simulink model "PARTAGE_last"  (Simulink 7.5)
settings: Solver=ode45  StartTime=0.0  StopTime=inf  RelTol=1e-3
settings Model: Creator=paris  LastModifiedBy=paris

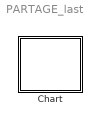
== system PARTAGE_last ==
  Chart : Stateflow chart  TreatAsAtomicUnit=on

== stateflow chart Chart ==
  state MODEL_ACTIVITE_SITUEE [parallel]
    settings: executionOrder=1
    state franchissement_VAG
      state Sortie_Virage
      state Fin_Gestion_Courbe
      state VAG_JAC_SVD
        state Entree_Virage
        state Approche_Virage
        state Debut_Gestion_Courbe
        MODEL_ACTIVITE_SITUEE.franchissement_VAG.VAG_JAC_SVD.Approche_Virage -> MODEL_ACTIVITE_SITUEE.franchissement_VAG.VAG_JAC_SVD.Entree_Virage : [ml.distPtA<=10]
        MODEL_ACTIVITE_SITUEE.franchissement_VAG.VAG_JAC_SVD.Entree_Virage -> MODEL_ACTIVITE_SITUEE.franchissement_VAG.VAG_JAC_SVD.Debut_Gestion_Courbe : [ml.distPtA<=0.01]
        (default) -> MODEL_ACTIVITE_SITUEE.franchissement_VAG.VAG_JAC_SVD.Approche_Virage
      state Pas_Code
      (junction 74) -> VAG_JAC_SVD [order 1] : [ml.distPtA<=50 && ml.distPtC>=0]
      MODEL_ACTIVITE_SITUEE.franchissement_VAG.Fin_Gestion_Courbe -> MODEL_ACTIVITE_SITUEE.franchissement_VAG.Sortie_Virage : [ml.distPtC<=0.01]
      MODEL_ACTIVITE_SITUEE.franchissement_VAG.VAG_JAC_SVD.Debut_Gestion_Courbe -> MODEL_ACTIVITE_SITUEE.franchissement_VAG.Fin_Gestion_Courbe : [ml.distPtB<=0.01]
      (junction 74) -> MODEL_ACTIVITE_SITUEE.franchissement_VAG.Pas_Code [order 2]
      (default) -> (junction 74)
    state Debut_Situation/
    state franchissement_VAD
      state Sortie_Virage
      state Fin_Gestion_Courbe
      state VAD_JAC_SVG
        state Entree_Virage
        state Approche_Virage
        state Debut_Gestion_Courbe
        MODEL_ACTIVITE_SITUEE.franchissement_VAD.VAD_JAC_SVG.Approche_Virage -> MODEL_ACTIVITE_SITUEE.franchissement_VAD.VAD_JAC_SVG.Entree_Virage : [ml.distPtA<=10]
        MODEL_ACTIVITE_SITUEE.franchissement_VAD.VAD_JAC_SVG.Entree_Virage -> MODEL_ACTIVITE_SITUEE.franchissement_VAD.VAD_JAC_SVG.Debut_Gestion_Courbe : [ml.distPtA<=0.01]
        (default) -> MODEL_ACTIVITE_SITUEE.franchissement_VAD.VAD_JAC_SVG.Approche_Virage
      state Pas_Code
      (junction 75) -> VAD_JAC_SVG [order 1] : [ml.distPtA<=50 && ml.distPtC>=0]
      MODEL_ACTIVITE_SITUEE.franchissement_VAD.Fin_Gestion_Courbe -> MODEL_ACTIVITE_SITUEE.franchissement_VAD.Sortie_Virage : [ml.distPtC<=0.01]
      MODEL_ACTIVITE_SITUEE.franchissement_VAD.VAD_JAC_SVG.Debut_Gestion_Courbe -> MODEL_ACTIVITE_SITUEE.franchissement_VAD.Fin_Gestion_Courbe : [ml.distPtB<=0.01]
      (junction 75) -> MODEL_ACTIVITE_SITUEE.franchissement_VAD.Pas_Code [order 2]
      (default) -> (junction 75)
    state Gestion_obstacle
      state Depassement
        state Approche
        state Imminent
        state Debut_Depassement
        state Fin_Depassement
        MODEL_ACTIVITE_SITUEE.Gestion_obstacle.Depassement.Approche -> MODEL_ACTIVITE_SITUEE.Gestion_obstacle.Depassement.Imminent [order 1] : [ml.cligno==-1]
        MODEL_ACTIVITE_SITUEE.Gestion_obstacle.Depassement.Approche -> Debut_Depassement [order 2] : [ml.progression_SV==1]
        MODEL_ACTIVITE_SITUEE.Gestion_obstacle.Depassement.Imminent -> Debut_Depassement : [ml.progression_SV==1]
        Debut_Depassement -> Fin_Depassement : [ml.etat_obstacle==0]
        (default) -> MODEL_ACTIVITE_SITUEE.Gestion_obstacle.Depassement.Approche
      state Approche_Obstacle
      state Gestion_Interaction_ContreSens
        state Debut_Interaction
        state Fin_Interaction
        state Approche
        state Imminent
        Debut_Interaction -> Fin_Interaction : [ml.etat_obstacle==0]
        MODEL_ACTIVITE_SITUEE.Gestion_obstacle.Gestion_Interaction_ContreSens.Approche -> MODEL_ACTIVITE_SITUEE.Gestion_obstacle.Gestion_Interaction_ContreSens.Imminent [order 1] : [ml.tlc<=1 || ml.ttc<=2]
        MODEL_ACTIVITE_SITUEE.Gestion_obstacle.Gestion_Interaction_ContreSens.Imminent -> Debut_Interaction : [ml.progression_SV==1]
        MODEL_ACTIVITE_SITUEE.Gestion_obstacle.Gestion_Interaction_ContreSens.Approche -> Debut_Interaction [order 2] : [ml.progression_SV==1]
      state Gestion_Obstacle_Fixe
        state Debut_Gestion_Obstacle
        state Fin_Gestion_Obstacle
        state Imminent
        state Approche
        Debut_Gestion_Obstacle -> Fin_Gestion_Obstacle : [ml.etat_obstacle==0]
        MODEL_ACTIVITE_SITUEE.Gestion_obstacle.Gestion_Obstacle_Fixe.Imminent -> Debut_Gestion_Obstacle : [ml.progression_SV==1]
        (default) -> MODEL_ACTIVITE_SITUEE.Gestion_obstacle.Gestion_Obstacle_Fixe.Approche
        MODEL_ACTIVITE_SITUEE.Gestion_obstacle.Gestion_Obstacle_Fixe.Approche -> Debut_Gestion_Obstacle [order 2] : [ml.progression_SV==1]
        MODEL_ACTIVITE_SITUEE.Gestion_obstacle.Gestion_Obstacle_Fixe.Approche -> MODEL_ACTIVITE_SITUEE.Gestion_obstacle.Gestion_Obstacle_Fixe.Imminent [order 1] : [ml.tlc<=1 || ml.ttc<=2]
      Approche_Obstacle -> Depassement [order 1] : [ml.sensCirculation_obstacle==21 || ml.type_obstacle==30]
      (default) -> Approche_Obstacle [order 2]
      Approche_Obstacle -> Gestion_Interaction_ContreSens [order 2] : [ml.sensCirculation_obstacle==22 && ml.type_obstacle<>30]
      (default) -> MODEL_ACTIVITE_SITUEE.Gestion_obstacle.Gestion_Interaction_ContreSens.Approche [order 1]
      Approche_Obstacle -> Gestion_Obstacle_Fixe [order 3] : [ml.sensCirculation==20]
    state Fin_Situation
    (default) -> Debut_Situation
    Debut_Situation -> franchissement_VAG [order 2] : [(ml.type_infrastructure==60 || ml.type_infrastructure==61)]
    (junction 73) -> Fin_Situation : [ml.type_infrastructure==62]
    Debut_Situation -> franchissement_VAD [order 3] : [ml.type_infrastructure==63 || ml.type_infrastructure==64]
    Debut_Situation -> Gestion_obstacle [order 1] : [ml.etat_obstacle>0]
    franchissement_VAD -> (junction 73)
    Fin_Situation -> Debut_Situation
    franchissement_VAG -> (junction 73)
    Fin_Depassement -> (junction 71)
    Fin_Interaction -> (junction 71)
    Fin_Gestion_Obstacle -> (junction 71)
    (junction 71) -> Fin_Situation : [ml.etat_obstacle==0]
    MODEL_ACTIVITE_SITUEE.franchissement_VAD.Sortie_Virage -> Fin_Situation
    MODEL_ACTIVITE_SITUEE.franchissement_VAG.Sortie_Virage -> Fin_Situation
  state MANOEUVRE_SV [parallel]
    settings: executionOrder=2
    state Conduite_Dans_Voie
    state SORTIE_VOIE
      state SVG
        state HORS_VOIE
          state Recentration
          state Excentration
          MANOEUVRE_SV.SORTIE_VOIE.SVG.HORS_VOIE.Excentration -> MANOEUVRE_SV.SORTIE_VOIE.SVG.HORS_VOIE.Recentration : [ml.progression_SV==-1]
        state RSV
        MANOEUVRE_SV.SORTIE_VOIE.SVG.RSV -> MANOEUVRE_SV.SORTIE_VOIE.SVG.HORS_VOIE.Excentration : [ml.progression_SV==1]
        (default) -> MANOEUVRE_SV.SORTIE_VOIE.SVG.RSV
      state SVD
        state HORS_VOIE
          state Recentration
          state Excentration
          MANOEUVRE_SV.SORTIE_VOIE.SVD.HORS_VOIE.Excentration -> MANOEUVRE_SV.SORTIE_VOIE.SVD.HORS_VOIE.Recentration : [ml.progression_SV==-1]
        state RSV
        (default) -> MANOEUVRE_SV.SORTIE_VOIE.SVD.RSV
        MANOEUVRE_SV.SORTIE_VOIE.SVD.RSV -> MANOEUVRE_SV.SORTIE_VOIE.SVD.HORS_VOIE.Excentration : [ml.progression_SV==1]
    (default) -> MANOEUVRE_SV.Conduite_Dans_Voie
    MANOEUVRE_SV.SORTIE_VOIE.SVD.HORS_VOIE.Recentration -> MANOEUVRE_SV.Conduite_Dans_Voie : [ml.etat_SV==0]
    MANOEUVRE_SV.Conduite_Dans_Voie -> SVD [order 2] : [ml.lateralisation_SV==1 && in(Risque_Sortie_Voie.SV_Imminente)]
    MANOEUVRE_SV.SORTIE_VOIE.SVG.HORS_VOIE.Recentration -> MANOEUVRE_SV.Conduite_Dans_Voie : [ml.etat_SV==0]
    MANOEUVRE_SV.Conduite_Dans_Voie -> SVG [order 1] : [ml.lateralisation_SV==-1 && in(Risque_Sortie_Voie.SV_Imminente)]
  state Jugement_Adequation_Comportement [parallel]
    settings: executionOrder=3
    state Defaut_Maitrise
    state Sortie_Voie_Legitime
    state Conduite_Dans_Voie
    state Optimisation_Trajectoire
    (junction 70) -> Optimisation_Trajectoire [order 3] : [in(MODEL_ACTIVITE_SITUEE.franchissement_VAG.VAG_JAC_SVD) && in(MANOEUVRE_SV.SORTIE_VOIE.SVD)]
    (default) -> Jugement_Adequation_Comportement.Conduite_Dans_Voie
    Jugement_Adequation_Comportement.Conduite_Dans_Voie -> (junction 70) : [in(Risque_Sortie_Voie.SV_Imminente) || in(Risque_Sortie_Voie.SV_Effective)]
    (junction 70) -> Optimisation_Trajectoire [order 5] : [in(MODEL_ACTIVITE_SITUEE.franchissement_VAD.VAD_JAC_SVG) && in(MANOEUVRE_SV.SORTIE_VOIE.SVG) ]
    (junction 70) -> Sortie_Voie_Legitime [order 1] : [ml.etat_obstacle==1]
    (junction 70) -> Optimisation_Trajectoire [order 2] : [(in(MODEL_ACTIVITE_SITUEE.franchissement_VAG.VAG_JAC_SVD) || in(MODEL_ACTIVITE_SITUEE.franchissement_VAG.Fin_Gestion_Courbe)) && in(MANOEUVRE_SV.SORTIE_VOIE.SVG)]
    (junction 70) -> Optimisation_Trajectoire [order 4] : [in(MODEL_ACTIVITE_SITUEE.franchissement_VAD) && in(MANOEUVRE_SV.SORTIE_VOIE.SVD)]
    Jugement_Adequation_Comportement -> Jugement_Adequation_Comportement.Conduite_Dans_Voie : [in(Risque_Sortie_Voie.Dans_Voie)]
    (junction 70) -> Defaut_Maitrise [order 6] : [ml.type_infrastructure<>62]
    Optimisation_Trajectoire -> Defaut_Maitrise : [ml.penteVolant<=-17 || ml.enfoncement_frein>=35 ]
  state Risque_Sortie_Voie [parallel]
    settings: executionOrder=4
    state SV_Imminente
    state SV_Possible
    state SV_Effective
    state Dans_Voie
    (default) -> Dans_Voie
    Dans_Voie -> SV_Possible : [abs(ml.tlc)<=3]
    SV_Possible -> SV_Imminente : [abs(ml.tlc)<=1.5]
    SV_Imminente -> SV_Effective : [abs(ml.progression_SV)==1]
    SV_Effective -> Dans_Voie : [ml.etat_SV==0]
  state Regles_Decisionnelles_Interaction_Homme_Machine [parallel]
    settings: executionOrder=5
    state Conduite_Dans_Voie
    state Aide_Requise
      state Aide_Maintien_Voie
      state Correction_Habitudes
    state Ne_Pas_Entraver_Activite
      state Legitime_NonCritique
      state Legitime_Critique
      (junction 72) -> Legitime_NonCritique [order 2] : [ml.lateralisation_SV==1 && ml.type_accotement==68]
      (junction 72) -> Legitime_NonCritique [order 1] : [ml.lateralisation_SV==1 && ml.type_accotement==69]
      (junction 72) -> Legitime_Critique [order 3] : [ml.lateralisation_SV==-1 && ml.marquage==67]
      (default) -> (junction 72)
      (junction 72) -> Legitime_Critique [order 4]
    (default) -> Regles_Decisionnelles_Interaction_Homme_Machine.Conduite_Dans_Voie
    Regles_Decisionnelles_Interaction_Homme_Machine -> Ne_Pas_Entraver_Activite [order 4] : [in(Jugement_Adequation_Comportement.Sortie_Voie_Legitime)]
    Regles_Decisionnelles_Interaction_Homme_Machine -> Regles_Decisionnelles_Interaction_Homme_Machine.Conduite_Dans_Voie [order 2] : [in(Jugement_Adequation_Comportement.Conduite_Dans_Voie) || ml.etat_SV==0]
    Regles_Decisionnelles_Interaction_Homme_Machine -> Aide_Maintien_Voie [order 1] : [in(Jugement_Adequation_Comportement.Defaut_Maitrise)]
    Regles_Decisionnelles_Interaction_Homme_Machine -> Correction_Habitudes [order 3] : [in(Jugement_Adequation_Comportement.Optimisation_Trajectoire)]
